simulink model "DisplayModel"  (R2013b)
settings: Solver=FixedStepDiscrete  StartTime=0.0  StopTime=500  FixedStep=1  RelTol=1e-3
PostLoadFcn:
  | clear all;
  | close all;
  | delete(get(0,'Children'));
  | load busdata.mat;
  | load Input_data.mat;
StartFcn:
  | delete(get(0,'Children'));
  | sfcockpitDisplay;
undefined symbols (not defined in the file): AirplaneDirection, AirSpeed, Altitude, APUData, Bearing, CabinPressure, delete, Distance, ECAMInput, EFIS_Pressure, EPR, ExhaustTemp, FlapPosition, FlightAttitude, FuelPressure, FuelQuantity, GroundSpeed, h_ECAM, h_EFIS, h_FCU, h_ND, h_ND_AD, h_PFD_Pages, h_WEng, HydraulicPressure, LandingGear, NDPageInput, OilPressure, RateOfTurn, RPM, SelectedHeading, Temperature, VerticalSpeed
libraries: CockpitDisplayLib x35, aerolibanimutils x1, simulink x1
(part 2 of 2)

== system DisplayModel/Control_and_Display_Logic/SignalConditioning/SignalSelection/DataValidityLandingGearRightLock/Range Threshold ==
  note: This test checks whether the signals are within
      | the normal bounds of the sensor
  signals : Inport
  Logical Operator : Logic  AllPortsSameDT=off
  Relational Operator : RelationalOperator  Operator=<
  Relational Operator1 : RelationalOperator  Operator=>
  pos_max : Constant  Value=1.5
  pos_min : Constant  Value=-0.5
  Validity : Outport
  wires:
  Logical Operator/1 -> Validity/1
  pos_min/1 -> Relational Operator1/2
  pos_max/1 -> Relational Operator/2
  Relational Operator1/1 -> Logical Operator/2
  Relational Operator/1 -> Logical Operator/1
  signals/1 -> Relational Operator1/1, Relational Operator/1

== system DisplayModel/Control_and_Display_Logic/SignalConditioning/SignalSelection/DataValidityLandingGearRightLock/Screen Signals ==
  signals : Inport
  Validity : Inport  Port=2
  Chart (MATLAB) : Stateflow chart  TreatAsAtomicUnit=on
  Data Type Conversion : DataTypeConversion  OutDataTypeStr=double
  validated sensor value : Outport
  wires:
  Chart (MATLAB)/1(valid_signal) -> validated sensor value/1
  Validity/1 -> Data Type Conversion/1
  signals/1 -> Chart (MATLAB)/1(signals)
  Data Type Conversion/1 -> Chart (MATLAB)/2(validity)

== system DisplayModel/Inputs/Sensors/SwitchedOff/LandingGearLeftLock_sensor/Sensor_DataConversion ==
  In1 : Inport
  Measured Speed1 : Subsystem
  Measured Speed2 : Subsystem
  Measured Speed3 : Subsystem
  Vector Concatenate : Concatenate  NumInputs=3
  Out1 : Outport
  wires:
  Measured Speed2/1(Out1) -> Vector Concatenate/2
  In1/1 -> Measured Speed2/1(position), Measured Speed1/1(in), Measured Speed3/1(position)
  Measured Speed3/1(Out1) -> Vector Concatenate/3
  Vector Concatenate/1 -> Out1/1  "RPM"
  Measured Speed1/1(Out) -> Vector Concatenate/1  "RPM"

== system DisplayModel/Inputs/Sensors/SwitchedOff/LandingGearRightLock_sensor/Sensor_DataConversion ==
  In1 : Inport
  Measured Speed1 : Subsystem
  Measured Speed2 : Subsystem
  Measured Speed3 : Subsystem
  Vector Concatenate : Concatenate  NumInputs=3
  Out1 : Outport
  wires:
  Measured Speed1/1(Out) -> Vector Concatenate/1  "RPM"
  Vector Concatenate/1 -> Out1/1  "RPM"
  Measured Speed3/1(Out1) -> Vector Concatenate/3
  In1/1 -> Measured Speed3/1(position), Measured Speed1/1(in), Measured Speed2/1(position)
  Measured Speed2/1(Out1) -> Vector Concatenate/2

== system DisplayModel/Inputs/Sensors/SwitchedOn/LandingGearLeftLock_sensor/Sensor_DataConversion ==
  In1 : Inport
  Measured Speed1 : Subsystem
  Measured Speed2 : Subsystem
  Measured Speed3 : Subsystem
  Vector Concatenate : Concatenate  NumInputs=3
  Out1 : Outport
  wires:
  Measured Speed2/1(Out1) -> Vector Concatenate/2
  In1/1 -> Measured Speed2/1(position), Measured Speed1/1(in), Measured Speed3/1(position)
  Measured Speed3/1(Out1) -> Vector Concatenate/3
  Vector Concatenate/1 -> Out1/1  "RPM"
  Measured Speed1/1(Out) -> Vector Concatenate/1  "RPM"

== system DisplayModel/Inputs/Sensors/SwitchedOn/LandingGearRightLock_sensor/Sensor_DataConversion ==
  In1 : Inport
  Measured Speed1 : Subsystem
  Measured Speed2 : Subsystem
  Measured Speed3 : Subsystem
  Vector Concatenate : Concatenate  NumInputs=3
  Out1 : Outport
  wires:
  Measured Speed1/1(Out) -> Vector Concatenate/1  "RPM"
  Vector Concatenate/1 -> Out1/1  "RPM"
  Measured Speed3/1(Out1) -> Vector Concatenate/3
  In1/1 -> Measured Speed3/1(position), Measured Speed1/1(in), Measured Speed2/1(position)
  Measured Speed2/1(Out1) -> Vector Concatenate/2

== system DisplayModel/Inputs/Sensors/SwitchedOff/LandingGearLeftLock_sensor/Sensor_DataConversion/Measured Speed1 ==
  in : Inport
  Out : Outport
  wires:
  in/1 -> Out/1

== system DisplayModel/Inputs/Sensors/SwitchedOff/LandingGearLeftLock_sensor/Sensor_DataConversion/Measured Speed2 ==
  position : Inport
  Out1 : Outport
  wires:
  position/1 -> Out1/1

== system DisplayModel/Inputs/Sensors/SwitchedOff/LandingGearLeftLock_sensor/Sensor_DataConversion/Measured Speed3 ==
  position : Inport
  Out1 : Outport
  wires:
  position/1 -> Out1/1

== system DisplayModel/Inputs/Sensors/SwitchedOff/LandingGearRightLock_sensor/Sensor_DataConversion/Measured Speed1 ==
  in : Inport
  Out : Outport
  wires:
  in/1 -> Out/1

== system DisplayModel/Inputs/Sensors/SwitchedOff/LandingGearRightLock_sensor/Sensor_DataConversion/Measured Speed2 ==
  position : Inport
  Out1 : Outport
  wires:
  position/1 -> Out1/1

== system DisplayModel/Inputs/Sensors/SwitchedOff/LandingGearRightLock_sensor/Sensor_DataConversion/Measured Speed3 ==
  position : Inport
  Out1 : Outport
  wires:
  position/1 -> Out1/1

== system DisplayModel/Inputs/Sensors/SwitchedOn/LandingGearLeftLock_sensor/Sensor_DataConversion/Measured Speed1 ==
  in : Inport
  Out : Outport
  wires:
  in/1 -> Out/1

== system DisplayModel/Inputs/Sensors/SwitchedOn/LandingGearLeftLock_sensor/Sensor_DataConversion/Measured Speed2 ==
  position : Inport
  Out1 : Outport
  wires:
  position/1 -> Out1/1

== system DisplayModel/Inputs/Sensors/SwitchedOn/LandingGearLeftLock_sensor/Sensor_DataConversion/Measured Speed3 ==
  position : Inport
  Out1 : Outport
  wires:
  position/1 -> Out1/1

== system DisplayModel/Inputs/Sensors/SwitchedOn/LandingGearRightLock_sensor/Sensor_DataConversion/Measured Speed1 ==
  in : Inport
  Out : Outport
  wires:
  in/1 -> Out/1

== system DisplayModel/Inputs/Sensors/SwitchedOn/LandingGearRightLock_sensor/Sensor_DataConversion/Measured Speed2 ==
  position : Inport
  Out1 : Outport
  wires:
  position/1 -> Out1/1

== system DisplayModel/Inputs/Sensors/SwitchedOn/LandingGearRightLock_sensor/Sensor_DataConversion/Measured Speed3 ==
  position : Inport
  Out1 : Outport
  wires:
  position/1 -> Out1/1

== stateflow chart DisplayModel/Control_and_Display_Logic/SignalConditioning/SignalSelection/DataValidityLandingGearRightLock/Screen Signals/Chart (MATLAB) ==
  state Screen
    note: no valid signals
    state three
      (default) -> (junction 112) : {sum_sig=signals(1)+signals(2)+signals(3);}
      (junction 112) -> (junction 114) : {middle=sum_sig - (max(signals) + min(signals));}
      (junction 114) -> (junction 113) [order 1] : [bad==1]
      (junction 113) -> (junction 116) : {none();}
      (junction 114) -> (junction 115) [order 2] : {valid_signal=logical(middle);}
      (junction 115) -> (junction 117)
      (junction 117) -> (junction 118) : {prev_signal=valid_signal;}
      (junction 118) -> (junction 119) : {count=0;}
    state zero
      (default) -> (junction 129) : {none();}
    state one
      note: Only one valid sensor - just use the valid signal.
          | Failure is false
      (default) -> (junction 102) : {valid_signal=signals(select(1));}
      (junction 102) -> (junction 103) : {prev_signal=valid_signal;}
      (junction 103) -> (junction 104) : {count=0;}
    state two
      (default) -> (junction 24) : {diff=abs(signals(select(1))-signals(select(2)));}
      (junction 24) -> (junction 23) [order 1] : [diff>diff_max]
      (junction 23) -> (junction 26) : {none();}
      (junction 24) -> (junction 25) [order 2] : {mean=(signals(select(1))+signals(select(2)))/2;}
      (junction 25) -> (junction 27) : {valid_signal=logical(mean);}
      (junction 27) -> (junction 28) : {prev_signal=valid_signal;}
      (junction 28) -> (junction 29) : {count=0;}
    (default) -> (junction 131) : {n=valid_sensors();bad = 0;}
    three -> Screen
    (junction 131) -> zero [order 4]
    (junction 131) -> three [order 1] : [n==3]
    zero -> Screen
    (junction 131) -> two [order 2] : [n==2]
    (junction 131) -> one [order 3] : [n==1]
    one -> Screen
    two -> Screen
  state none [function]
    (default) -> (junction 2)
    (junction 2) -> (junction 3) : {count=count+1;}
    (junction 3) -> (junction 4) [order 1] : [count>3]
    (junction 4) -> (junction 5) : {count=3;}
    (junction 5) -> (junction 6) : {valid_signal=false;}
    (junction 3) -> (junction 7) [order 2] : {valid_signal=prev_signal;}
    (junction 6) -> (junction 9)
    (junction 7) -> (junction 8)
    (junction 8) -> (junction 9)
  (default) -> Screen : {bad = 0;count = 0;prev_signal = false;}
  data: middle local double; diff local double; mean local double; num function_output double size=1; signals input boolean size=3; prev_signal local boolean size=1; count local double size=1; diff_max constant double =3; bad local double size=1; validity input; valid_signal output boolean size=1; sum_sig local double size=1; n local; select local double size=2
  function num = valid_sensors:
    | function num = valid_sensors
    | 
    | aVarTruthTableCondition_1 = false;
    | aVarTruthTableCondition_2 = false;
    | aVarTruthTableCondition_3 = false;
    | 
    | 
    | 
    | aVarTruthTableCondition_1 = logical(validity(1) == 1);
    | 
    | 
    | aVarTruthTableCondition_2 = logical(validity(2) == 1);
    | 
    | 
    | aVarTruthTableCondition_3 = logical(validity(3) == 1);
    | 
    | if (aVarTruthTableCondition_1 && aVarTruthTableCondition_2 && aVarTruthTableCondition_3)
    |     aFcnTruthTableAction_1();
    | elseif (aVarTruthTableCondition_1 && aVarTruthTableCondition_2 && ~aVarTruthTableCondition_3)
    |     aFcnTruthTableAction_2();
    | elseif (aVarTruthTableCondition_1 && ~aVarTruthTableCondition_2 && aVarTruthTableCondition_3)
    |     aFcnTruthTableAction_3();
    | elseif (aVarTruthTableCondition_1 && ~aVarTruthTableCondition_2 && ~aVarTruthTableCondition_3)
    |     aFcnTruthTableAction_5();
    | elseif (~aVarTruthTableCondition_1 && aVarTruthTableCondition_2 && aVarTruthTableCondition_3)
    |     aFcnTruthTableAction_4();
    | elseif (~aVarTruthTableCondition_1 && aVarTruthTableCondition_2 && ~aVarTruthTableCondition_3)
    |     aFcnTruthTableAction_6();
    | elseif (~aVarTruthTableCondition_1 && ~aVarTruthTableCondition_2 && aVarTruthTableCondition_3)
    |     aFcnTruthTableAction_7();
    | else % Default
    |     None();
    | end
    | 
    | function aFcnTruthTableAction_1()
    | 
    | % All 3 signals valid
    | 
    | num = 3;
    | 
    | function aFcnTruthTableAction_2()
    | 
    | % Signals 1&2 valid
    | 
    | num = 2;
    | select(1)=1;
    | select(2)=2;
    | 
    | function aFcnTruthTableAction_3()
    | 
    | % Signals 1&3 valid
    | 
    | num = 2;
    | select(1)=1;
    | select(2)=3;
    | 
    | function aFcnTruthTableAction_4()
    | 
    | % Signals 2&3 valid
    | 
    | num = 2;
    | select(1)=2;
    | select(2)=3;
    | 
    | function aFcnTruthTableAction_5()
    | 
    | % Signal 1 valid
    | 
    | num = 1;
    | select(1)=1;
    | select(2)=0;
    | 
    | function aFcnTruthTableAction_6()
    | 
    | % Signal 2 valid
    | 
    | num = 1;
    | select(1)=2;
    | select(2)=0;
    | 
    | function aFcnTruthTableAction_7()
    | 
    | % Signal 3 valid
    | 
    | num = 1;
    | select(1)=3;
    | select(2)=0;
    | 
    | function None()
    | 
    | % no signals valid
    | 
    | num = 0;

== stateflow chart DisplayModel/Inputs/UserSelection/EnergyManagement/EnergyManagement ==
  state APU_LOGIC [parallel]
    settings: executionOrder=1
    state OFF
      entry: APU_Mode = 0;
    state APU_PrepareForStart
      entry: APU_Mode = 1;
    state APU_Start
    state APU_Running
      entry: APU_Mode = 2;
    (default) -> APU_LOGIC.OFF
    APU_LOGIC.OFF -> APU_PrepareForStart : [APU_MasterSwitch]
    APU_PrepareForStart -> APU_Start : [APU_StartSwitch]
    APU_Start -> APU_Running : after(5,sec)
  state Engine_LOGIC [parallel]
    settings: executionOrder=2
    state OFF
    state Engine_PrepareForStart
      entry:Engine_Mode = 1;
    state Engine_Start
    state Engine_Running
      entry:Engine_Mode = 2;
    (default) -> Engine_LOGIC.OFF
    Engine_LOGIC.OFF -> Engine_PrepareForStart : [APU_Mode ==2 && Engine_MasterSwitch]
    Engine_PrepareForStart -> Engine_Start : [Engine_StartSwitch]
    Engine_Start -> Engine_Running : after(5,sec)
  data: APU_Mode output; APU_MasterSwitch input; APU_StartSwitch input; Engine_MasterSwitch input; Engine_StartSwitch input; Engine_Mode output

== stateflow chart DisplayModel/Control_and_Display_Logic/SignalConditioning/SignalSelection/DataValidityLandingGearLeftLock/Screen Signals/Chart (MATLAB) ==
  state Screen
    note: no valid signals
    state three
      (default) -> (junction 112) : {sum_sig=signals(1)+signals(2)+signals(3);}
      (junction 112) -> (junction 114) : {middle=sum_sig - (max(signals) + min(signals));}
      (junction 114) -> (junction 113) [order 1] : [bad==1]
      (junction 113) -> (junction 116) : {none();}
      (junction 114) -> (junction 115) [order 2] : {valid_signal=logical(middle);}
      (junction 115) -> (junction 117)
      (junction 117) -> (junction 118) : {prev_signal=valid_signal;}
      (junction 118) -> (junction 119) : {count=0;}
    state zero
      (default) -> (junction 129) : {none();}
    state one
      note: Only one valid sensor - just use the valid signal.
          | Failure is false
      (default) -> (junction 102) : {valid_signal=signals(select(1));}
      (junction 102) -> (junction 103) : {prev_signal=valid_signal;}
      (junction 103) -> (junction 104) : {count=0;}
    state two
      (default) -> (junction 24) : {diff=abs(signals(select(1))-signals(select(2)));}
      (junction 24) -> (junction 23) [order 1] : [diff>diff_max]
      (junction 23) -> (junction 26) : {none();}
      (junction 24) -> (junction 25) [order 2] : {mean=(signals(select(1))+signals(select(2)))/2;}
      (junction 25) -> (junction 27) : {valid_signal=logical(mean);}
      (junction 27) -> (junction 28) : {prev_signal=valid_signal;}
      (junction 28) -> (junction 29) : {count=0;}
    (default) -> (junction 131) : {n=valid_sensors();bad = 0;}
    three -> Screen
    (junction 131) -> zero [order 4]
    (junction 131) -> three [order 1] : [n==3]
    zero -> Screen
    (junction 131) -> two [order 2] : [n==2]
    (junction 131) -> one [order 3] : [n==1]
    one -> Screen
    two -> Screen
  state none [function]
    (default) -> (junction 2)
    (junction 2) -> (junction 3) : {count=count+1;}
    (junction 3) -> (junction 4) [order 1] : [count>3]
    (junction 4) -> (junction 5) : {count=3;}
    (junction 5) -> (junction 6) : {valid_signal=false;}
    (junction 3) -> (junction 7) [order 2] : {valid_signal=prev_signal;}
    (junction 6) -> (junction 9)
    (junction 7) -> (junction 8)
    (junction 8) -> (junction 9)
  (default) -> Screen : {bad = 0;count = 0;prev_signal = false;}
  data: middle local double; diff local double; mean local double; num function_output double size=1; signals input boolean size=3; prev_signal local boolean size=1; count local double size=1; diff_max constant double =3; bad local double size=1; validity input; valid_signal output boolean size=1; sum_sig local double size=1; n local; select local double size=2
  function num = valid_sensors:
    | function num = valid_sensors
    | 
    | aVarTruthTableCondition_1 = false;
    | aVarTruthTableCondition_2 = false;
    | aVarTruthTableCondition_3 = false;
    | 
    | 
    | 
    | aVarTruthTableCondition_1 = logical(validity(1) == 1);
    | 
    | 
    | aVarTruthTableCondition_2 = logical(validity(2) == 1);
    | 
    | 
    | aVarTruthTableCondition_3 = logical(validity(3) == 1);
    | 
    | if (aVarTruthTableCondition_1 && aVarTruthTableCondition_2 && aVarTruthTableCondition_3)
    |     aFcnTruthTableAction_1();
    | elseif (aVarTruthTableCondition_1 && aVarTruthTableCondition_2 && ~aVarTruthTableCondition_3)
    |     aFcnTruthTableAction_2();
    | elseif (aVarTruthTableCondition_1 && ~aVarTruthTableCondition_2 && aVarTruthTableCondition_3)
    |     aFcnTruthTableAction_3();
    | elseif (aVarTruthTableCondition_1 && ~aVarTruthTableCondition_2 && ~aVarTruthTableCondition_3)
    |     aFcnTruthTableAction_5();
    | elseif (~aVarTruthTableCondition_1 && aVarTruthTableCondition_2 && aVarTruthTableCondition_3)
    |     aFcnTruthTableAction_4();
    | elseif (~aVarTruthTableCondition_1 && aVarTruthTableCondition_2 && ~aVarTruthTableCondition_3)
    |     aFcnTruthTableAction_6();
    | elseif (~aVarTruthTableCondition_1 && ~aVarTruthTableCondition_2 && aVarTruthTableCondition_3)
    |     aFcnTruthTableAction_7();
    | else % Default
    |     None();
    | end
    | 
    | function aFcnTruthTableAction_1()
    | 
    | % All 3 signals valid
    | 
    | num = 3;
    | 
    | function aFcnTruthTableAction_2()
    | 
    | % Signals 1&2 valid
    | 
    | num = 2;
    | select(1)=1;
    | select(2)=2;
    | 
    | function aFcnTruthTableAction_3()
    | 
    | % Signals 1&3 valid
    | 
    | num = 2;
    | select(1)=1;
    | select(2)=3;
    | 
    | function aFcnTruthTableAction_4()
    | 
    | % Signals 2&3 valid
    | 
    | num = 2;
    | select(1)=2;
    | select(2)=3;
    | 
    | function aFcnTruthTableAction_5()
    | 
    | % Signal 1 valid
    | 
    | num = 1;
    | select(1)=1;
    | select(2)=0;
    | 
    | function aFcnTruthTableAction_6()
    | 
    | % Signal 2 valid
    | 
    | num = 1;
    | select(1)=2;
    | select(2)=0;
    | 
    | function aFcnTruthTableAction_7()
    | 
    | % Signal 3 valid
    | 
    | num = 1;
    | select(1)=3;
    | select(2)=0;
    | 
    | function None()
    | 
    | % no signals valid
    | 
    | num = 0;
